simulink model "DoubleTankSim_NonLinearCtrl"  (R2025b)
settings: Solver=VariableStepAuto  StartTime=0.0  StopTime=1500  RelTol=1e-3
values from neighbouring files (symbols this model uses):
  a_1 = 0.15025    [LabC.m]
  a_2 = 0.15615    [LabC.m]
  At = 33    [LabC.m]
  g = 981    [LabC.m]
  h_0 = 3.2    [LabC.m]
  Kd = 2*omega_n    (= 0.666666666667)    [LabC.m]
  Ki = 0.00005    (= 5e-05)    [LabC.m]
  Kp = omega_n^2    (= 0.111111111111)    [LabC.m]
  Q = [variance 0 0 ... (first row only)    [LabC.m]
  R = 0.1    [LabC.m]
  Ts = 0.02    [LabC.m]
  variance = 1e-8    (= 1e-08)    [LabC.m]
libraries: simulink x4, slpidlib x1
settings Model: Creator=kaspe  LastModifiedBy=William

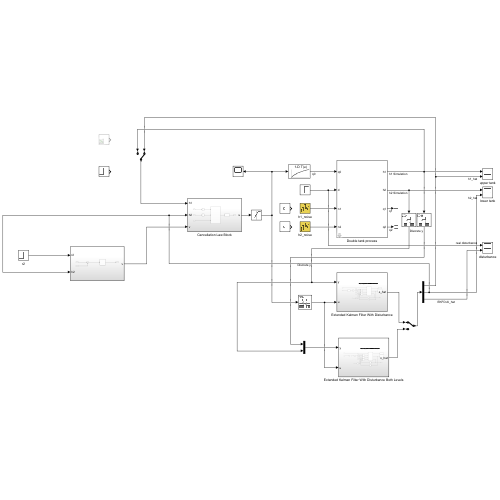
[thumbnail: Simulink's stored preview of the top-level diagram]
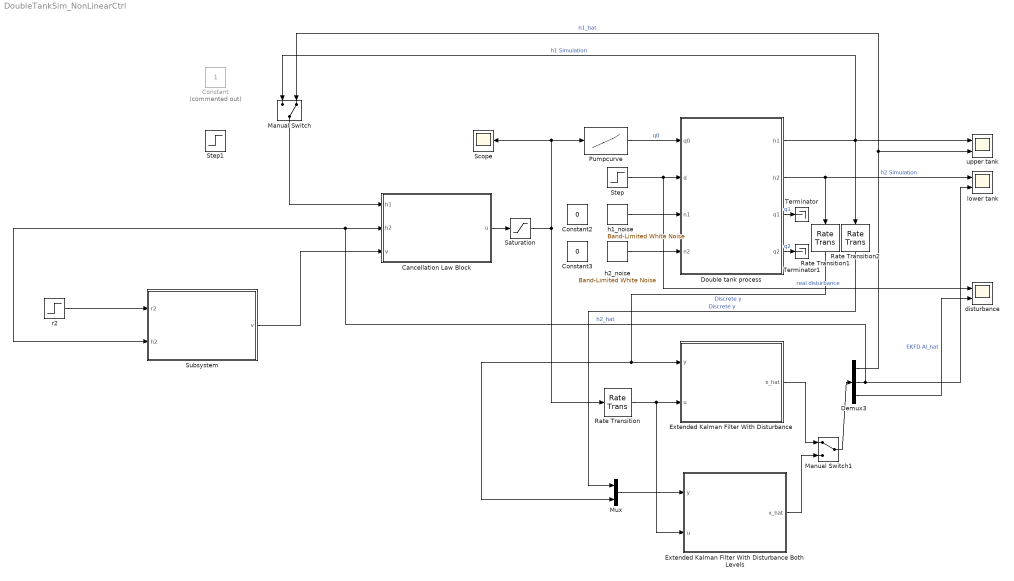
== system DoubleTankSim_NonLinearCtrl ==
  Cancellation Law Block : Subsystem
  Constant : Constant  Commented=on
  Constant2 : Constant  Value=0
  Constant3 : Constant  Value=0
  Demux3 : Demux  Outputs=3
  Double tank process : Subsystem  mask{At=33, a_1=0.151, a_2=0.16, hmax=15.5}
      mask prompts: At "Tank area (cm^2)"; a_1 "Upper tank opening area (cm^2)"; a_2 "Lower tank opening area (cm^2)"; hmax "Tank height (cm)"
      mask help: Double tank process parameters
  Extended Kalman Filter With Disturbance : Subsystem
  Extended Kalman Filter With Disturbance Both Levels : Subsystem
  Manual Switch : ManualSwitch  CurrentSetting=0
  Manual Switch1 : ManualSwitch
  Mux : Mux  Inputs=2
  Pumpcurve : Lookup_n-D  NumberOfTableDimensions=1  BreakpointsForDimension1=x  BreakpointsForDimension2=[1:3]  Table=y  RndMeth=Simplest  mask{x=[0.5,1,1.5,2,2.5,3,3.5,5,8,10], y=[16.47,20.75,24.52,27.63,30.06,32.49,34.80,40.28,48.24,52.43]}
      mask prompts: x "Values on x-axis"; y "Values on y-axis"
  Rate Transition : RateTransition  OutPortSampleTime=Ts
  Rate Transition1 : RateTransition  OutPortSampleTime=Ts
  Rate Transition2 : RateTransition  OutPortSampleTime=Ts
  Saturation : Saturate  UpperLimit=10  LowerLimit=0
  Scope : Scope
      settings: ActiveDisplayYMinimum=-1.2499999999999998  ActiveDisplayYMaximum=11.25  DataLoggingVariableName=ScopeData3
  Step : Step  Time=900  After=0.1  SampleTime=0
  Step1 : Step  Time=750  Before=1  After=1.25  SampleTime=0
  Subsystem : Subsystem
  Terminator : Terminator
  Terminator1 : Terminator
  disturbance : Scope  NumInputPorts=2
      settings: ActiveDisplayYMinimum=-1  ActiveDisplayYMaximum=1  DataLoggingVariableName=ScopeData2
  h1_noise : simulink/Sources/Band-Limited White Noise  Cov=[variance]  Ts=Ts  seed=[23342]
  h2_noise : simulink/Sources/Band-Limited White Noise  Cov=[variance]  Ts=Ts  seed=[23341]
  lower tank : Scope  NumInputPorts=2
      settings: ActiveDisplayYMinimum=-1.517228382859021  ActiveDisplayYMaximum=13.607589492730195
  r2 : Step  Time=500  Before=8  After=12  SampleTime=0
  upper tank : Scope  NumInputPorts=2
      settings: ActiveDisplayYMinimum=-1.986368348644401  ActiveDisplayYMaximum=17.525078273134039
  wires:
  Extended Kalman Filter With Disturbance/1(x_hat) -> Manual Switch1/1
  Pumpcurve/1 -> Double tank process/1(q0)  "q0"
  Double tank process/1(h1) -> upper tank/1, Manual Switch/1, Rate Transition2/1  "h1 Simulation"
  Step/1 -> Double tank process/2(d), disturbance/1  "real disturbance"
  h1_noise/1 -> Double tank process/3(n1)
  h2_noise/1 -> Double tank process/4(n2)
  Demux3/1 -> upper tank/2, Manual Switch/2  "h1_hat"
  Double tank process/2(h2) -> lower tank/1, Rate Transition1/1  "h2 Simulation"
  Demux3/2 -> Cancellation Law Block/2(h2), Subsystem/2(h2), lower tank/2  "h2_hat"
  Demux3/3 -> disturbance/2  "EKFD Al_hat"
  Rate Transition1/1 -> Extended Kalman Filter With Disturbance/1(y), Mux/2  "Discrete y"
  Rate Transition/1 -> Extended Kalman Filter With Disturbance/2(u), Extended Kalman Filter With Disturbance Both Levels/2(u)
  Double tank process/3(q1) -> Terminator/1  "q1"
  Double tank process/4(q2) -> Terminator1/1  "q2"
  Subsystem/1(v) -> Cancellation Law Block/3(v)
  Manual Switch/1 -> Cancellation Law Block/1(h1)
  r2/1 -> Subsystem/1(r2)
  Cancellation Law Block/1(u) -> Saturation/1
  Saturation/1 -> Scope/1, Pumpcurve/1, Rate Transition/1
  Mux/1 -> Extended Kalman Filter With Disturbance Both Levels/1(y)
  Rate Transition2/1 -> Mux/1  "Discrete y"
  Extended Kalman Filter With Disturbance Both Levels/1(x_hat) -> Manual Switch1/2
  Manual Switch1/1 -> Demux3/1

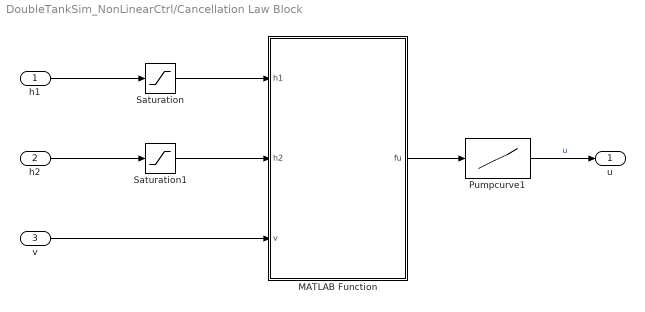
== system DoubleTankSim_NonLinearCtrl/Cancellation Law Block ==
  h1 : Inport
  h2 : Inport  Port=2
  v : Inport  Port=3
  MATLAB Function : MATLAB Function  TreatAsAtomicUnit=on
  Pumpcurve1 : Lookup_n-D  NumberOfTableDimensions=1  BreakpointsForDimension1=x  BreakpointsForDimension2=[1:3]  Table=y  RndMeth=Simplest  mask{x=[16.47,20.75,24.52,27.63,30.06,32.49,34.80,40.28,48.24,52.43], y=[0.5,1,1.5,2,2.5,3,3.5,5,8,10]}
      mask prompts: x "Values on x-axis"; y "Values on y-axis"
  Saturation : Saturate  UpperLimit=15.5  LowerLimit=0.001
  Saturation1 : Saturate  UpperLimit=15.5  LowerLimit=0.001
  u : Outport
  wires:
  MATLAB Function/1(fu) -> Pumpcurve1/1
  h1/1 -> Saturation/1
  h2/1 -> Saturation1/1
  Pumpcurve1/1 -> u/1  "u"
  v/1 -> MATLAB Function/3(v)
  Saturation/1 -> MATLAB Function/1(h1)
  Saturation1/1 -> MATLAB Function/2(h2)

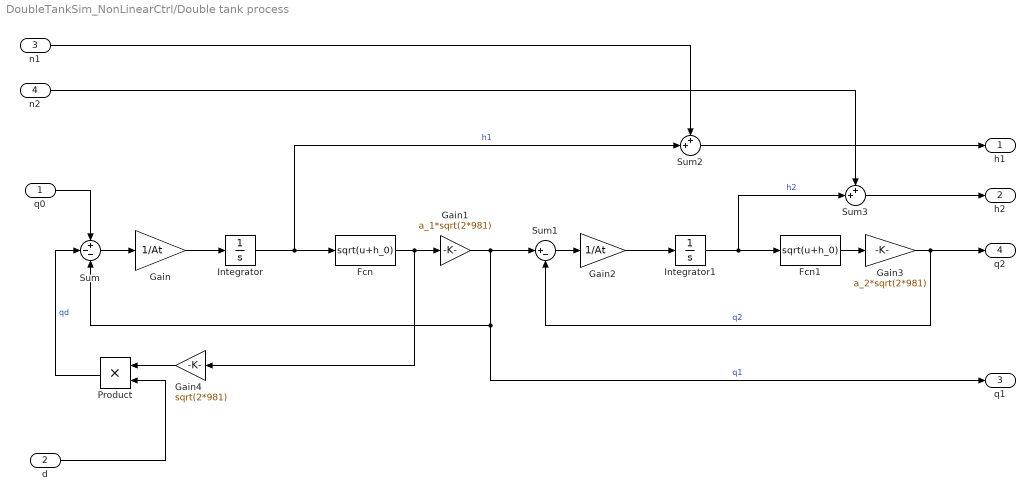
== system DoubleTankSim_NonLinearCtrl/Double tank process ==
  q0 : Inport
  d : Inport  Port=2
  n1 : Inport  Port=3
  n2 : Inport  Port=4
  Fcn : Fcn  Expr=sqrt(u+h_0)
  Fcn1 : Fcn  Expr=sqrt(u+h_0)
  Gain : Gain  Gain=1/At
  Gain1 : Gain  Gain=a_1*sqrt(2*981)
  Gain2 : Gain  Gain=1/At
  Gain3 : Gain  Gain=a_2*sqrt(2*981)
  Gain4 : Gain  Gain=sqrt(2*981)
  Integrator : Integrator  LimitOutput=on  UpperSaturationLimit=hmax  LowerSaturationLimit=0
  Integrator1 : Integrator  LimitOutput=on  UpperSaturationLimit=hmax  LowerSaturationLimit=0
  Product : Product  RndMeth=Zero
  Sum : Sum  Inputs=+--
  Sum1 : Sum  Inputs=|+-
  Sum2 : Sum  Inputs=++|
  Sum3 : Sum  Inputs=++|
  h1 : Outport  VectorParamsAs1DForOutWhenUnconnected=off
  h2 : Outport  Port=2  VectorParamsAs1DForOutWhenUnconnected=off
  q1 : Outport  Port=3  VectorParamsAs1DForOutWhenUnconnected=off
  q2 : Outport  Port=4  VectorParamsAs1DForOutWhenUnconnected=off
  wires:
  Sum/1 -> Gain/1
  Gain/1 -> Integrator/1
  Fcn/1 -> Gain4/1, Gain1/1
  Gain1/1 -> Sum1/1, q1/1, Sum/3  "q1"
  Sum1/1 -> Gain2/1
  Gain2/1 -> Integrator1/1
  Fcn1/1 -> Gain3/1
  Gain3/1 -> Sum1/2, q2/1  "q2"
  q0/1 -> Sum/1
  Integrator/1 -> Sum2/2, Fcn/1  "h1"
  Product/1 -> Sum/2  "qd"
  Integrator1/1 -> Sum3/2, Fcn1/1  "h2"
  d/1 -> Product/2
  Sum2/1 -> h1/1
  n1/1 -> Sum2/1
  Sum3/1 -> h2/1
  n2/1 -> Sum3/1
  Gain4/1 -> Product/1

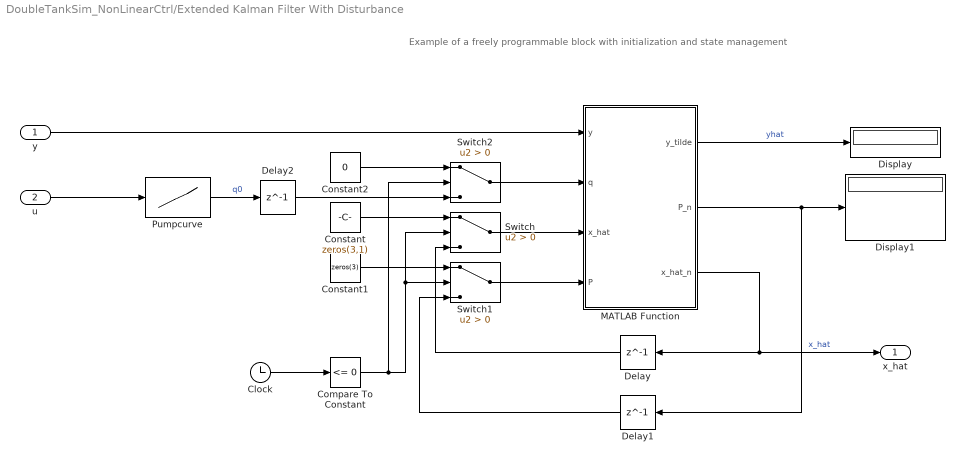
== system DoubleTankSim_NonLinearCtrl/Extended Kalman Filter With Disturbance ==
  note: Example of a freely programmable block with initialization and state management
  y : Inport
  u : Inport  Port=2
  Clock : Clock
  Compare To Constant : simulink/Logic and Bit Operations/Compare To Constant  relop=<=  const=0  OutDataTypeStr=boolean
  Constant : Constant  Value=zeros(3,1)
  Constant1 : Constant  Value=zeros(3)
  Constant2 : Constant  Value=0
  Delay : Delay  DelayLength=1  InitialCondition=0
  Delay1 : Delay  DelayLength=1  InitialCondition=0
  Delay2 : Delay  DelayLength=1  InitialCondition=0
  Display : Display
  Display1 : Display
  MATLAB Function : MATLAB Function  TreatAsAtomicUnit=on
  Pumpcurve : Lookup_n-D  NumberOfTableDimensions=1  BreakpointsForDimension1=x  BreakpointsForDimension2=[1:3]  Table=y  RndMeth=Simplest  mask{x=[0.5,1,1.5,2,2.5,3,3.5,5,8,10], y=[16.47,20.75,24.52,27.63,30.06,32.49,34.80,40.28,48.24,52.43]}
      mask prompts: x "Values on x-axis"; y "Values on y-axis"
  Switch : Switch  Criteria=u2 > Threshold  SaturateOnIntegerOverflow=off  InputSameDT=off
  Switch1 : Switch  Criteria=u2 > Threshold  SaturateOnIntegerOverflow=off  InputSameDT=off
  Switch2 : Switch  Criteria=u2 > Threshold  SaturateOnIntegerOverflow=off  InputSameDT=off
  x_hat : Outport  PortDimensions=3
  wires:
  Delay/1 -> Switch/3
  Switch/1 -> MATLAB Function/3(x_hat)
  Constant1/1 -> Switch1/1
  Compare To Constant/1 -> Switch2/2, Switch/2, Switch1/2
  Constant/1 -> Switch/1
  MATLAB Function/1(y_tilde) -> Display/1  "yhat"
  MATLAB Function/2(P_n) -> Delay1/1, Display1/1
  Clock/1 -> Compare To Constant/1
  Switch1/1 -> MATLAB Function/4(P)
  y/1 -> MATLAB Function/1(y)
  Delay1/1 -> Switch1/3
  Switch2/1 -> MATLAB Function/2(q)
  Constant2/1 -> Switch2/1
  Delay2/1 -> Switch2/3
  Pumpcurve/1 -> Delay2/1  "q0"
  u/1 -> Pumpcurve/1
  MATLAB Function/3(x_hat_n) -> Delay/1, x_hat/1  "x_hat"

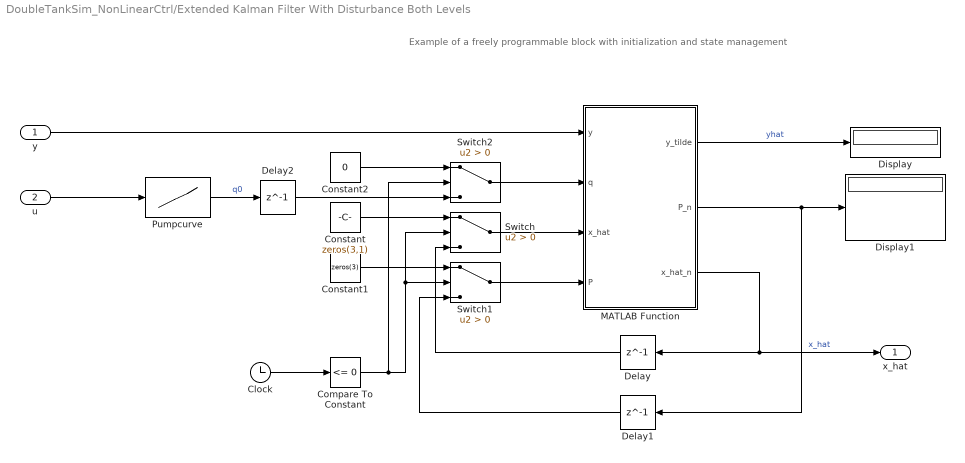
== system DoubleTankSim_NonLinearCtrl/Extended Kalman Filter With Disturbance Both Levels ==
  note: Example of a freely programmable block with initialization and state management
  y : Inport
  u : Inport  Port=2
  Clock : Clock
  Compare To Constant : simulink/Logic and Bit Operations/Compare To Constant  relop=<=  const=0  OutDataTypeStr=boolean
  Constant : Constant  Value=zeros(3,1)
  Constant1 : Constant  Value=zeros(3)
  Constant2 : Constant  Value=0
  Delay : Delay  DelayLength=1  InitialCondition=0
  Delay1 : Delay  DelayLength=1  InitialCondition=0
  Delay2 : Delay  DelayLength=1  InitialCondition=0
  Display : Display
  Display1 : Display
  MATLAB Function : MATLAB Function  TreatAsAtomicUnit=on
  Pumpcurve : Lookup_n-D  NumberOfTableDimensions=1  BreakpointsForDimension1=x  BreakpointsForDimension2=[1:3]  Table=y  RndMeth=Simplest  mask{x=[0.5,1,1.5,2,2.5,3,3.5,5,8,10], y=[16.47,20.75,24.52,27.63,30.06,32.49,34.80,40.28,48.24,52.43]}
      mask prompts: x "Values on x-axis"; y "Values on y-axis"
  Switch : Switch  Criteria=u2 > Threshold  SaturateOnIntegerOverflow=off  InputSameDT=off
  Switch1 : Switch  Criteria=u2 > Threshold  SaturateOnIntegerOverflow=off  InputSameDT=off
  Switch2 : Switch  Criteria=u2 > Threshold  SaturateOnIntegerOverflow=off  InputSameDT=off
  x_hat : Outport  PortDimensions=3
  wires:
  Delay/1 -> Switch/3
  Switch/1 -> MATLAB Function/3(x_hat)
  Constant1/1 -> Switch1/1
  Compare To Constant/1 -> Switch2/2, Switch/2, Switch1/2
  Constant/1 -> Switch/1
  MATLAB Function/1(y_tilde) -> Display/1  "yhat"
  MATLAB Function/2(P_n) -> Delay1/1, Display1/1
  Clock/1 -> Compare To Constant/1
  Switch1/1 -> MATLAB Function/4(P)
  y/1 -> MATLAB Function/1(y)
  Delay1/1 -> Switch1/3
  Switch2/1 -> MATLAB Function/2(q)
  Constant2/1 -> Switch2/1
  Delay2/1 -> Switch2/3
  Pumpcurve/1 -> Delay2/1  "q0"
  u/1 -> Pumpcurve/1
  MATLAB Function/3(x_hat_n) -> Delay/1, x_hat/1  "x_hat"

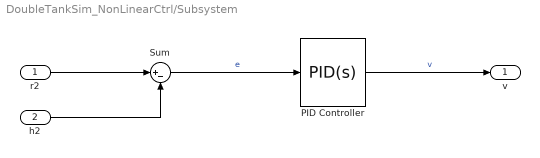
== system DoubleTankSim_NonLinearCtrl/Subsystem ==
  r2 : Inport
  h2 : Inport  Port=2
  PID Controller : slpidlib/PID Controller  Controller=PID  Form=Parallel  TimeDomain=Continuous-time  UseExternalTs=off  SampleTime=-1  IntegratorMethod=Forward Euler  FilterMethod=Forward Euler  ControllerParametersSource=internal  P=Kp  I=Ki  UseKiTs=off  D=Kd  UseExternalDerivativeSource=off  N=1  UseFilter=on  TunerSelectOption=Transfer Function Based (PID Tuner App)  InitialConditionSource=internal  InitialConditionForIntegrator=0  InitialConditionForFilter=0  DifferentiatorICPrevScaledInput=0  ExternalReset=none  TrackingMode=off  Kt=1  LimitOutput=off  SatLimitsSource=internal  UpperSaturationLimit=inf  LowerSaturationLimit=-inf  LinearizeAsGain=on  AntiWindupMode=none  Kb=1  LimitIntegrator=off  UpperIntegratorSaturationLimit=inf  LowerIntegratorSaturationLimit=-inf  POutMin=[]  POutMax=[]  IOutMin=[]  IOutMax=[]  DOutMin=[]  DOutMax=[]  NOutMin=[]  NOutMax=[]  SumOutMin=[]  SumOutMax=[]  SaturationOutMin=[]  SaturationOutMax=[]  PParamMin=[]  PParamMax=[]  IParamMin=[]  IParamMax=[]  DParamMin=[]  DParamMax=[]  NParamMin=[]  NParamMax=[]  KbParamMin=[]  KbParamMax=[]  KtParamMin=[]  KtParamMax=[]  KbOutMin=[]  KbOutMax=[]  KtOutMin=[]  KtOutMax=[]  IntegratorOutMin=[]  IntegratorOutMax=[]  FilterOutMin=[]  FilterOutMax=[]  SumI1OutMin=[]  SumI1OutMax=[]  SumI2OutMin=[]  SumI2OutMax=[]  SumI3OutMin=[]  SumI3OutMax=[]  SumI4OutMin=[]  SumI4OutMax=[]  SumDOutMin=[]  SumDOutMax=[]  DifferentiatorOutMin=[]  DifferentiatorOutMax=[]  FilterDiffOutCoefMin=[]  FilterDiffOutCoefMax=[]  ReciprocalOutMin=[]  ReciprocalOutMax=[]  SumDenOutMin=[]  SumDenOutMax=[]  SumNumOutMin=[]  SumNumOutMax=[]  DivideOutMin=[]  DivideOutMax=[]  UdiffTsProdOutMin=[]  UdiffTsProdOutMax=[]  NTsProdOutMin=[]  NTsProdOutMax=[]  UintegralTsProdOutMin=[]  UintegralTsProdOutMax=[]  UngainTsProdOutMin=[]  UngainTsProdOutMax=[]  ClampingZeroOutDataTypeStr=Inherit: Inherit via back propagation  ClampingZeroOutMin=[]  ClampingZeroOutMax=[]  FilterDenConstantOutDataTypeStr=Inherit: Inherit via back propagation  FilterDenConstantOutMin=[]  FilterDenConstantOutMax=[]  PCopyOutDataTypeStr=Inherit: Inherit via back propagation  PCopyOutMin=[]  PCopyOutMax=[]  NCopyOutDataTypeStr=Inherit: Inherit via back propagation  NCopyOutMin=[]  NCopyOutMax=[]  IntegratorContinuousStateAttributes=''  IntegratorStateMustResolveToSignalObject=off  IntegratorRTWStateStorageClass=Auto  FilterContinuousStateAttributes=''  FilterStateMustResolveToSignalObject=off  FilterRTWStateStorageClass=Auto  ParallelPVariant=InternalParameters  IdealPVariant=Disabled  IVariant=InternalParameters  DVariant=InternalParameters  IntegratorVariant=Continuous  SatVariant=Disabled  AWVariant=Passthrough  PCopyVariant=Disabled  TRVariant=Disabled  FdbkBlocksVariant=Forward  IdealPFdbkVariant=Disabled  SatFdbkVariant=Disabled  DerivativeFilterVariant=ContFilter  NVariant=InternalParameters  NCopyVariant=Disabled  FilterICVariant=InternalICsFilter  IntegratorICVariant=InternalICs  ExternalResetVariant=Disabled  TRSumVariant=Passthrough  SumFdbkVariant=Disabled  SumVariant=Sum_PID  TsampFilterVariant=InternalTs  TsampNgainVariant=Passthrough  TsampIntegralVariant=Disabled_SignalSpec  ExternalSaturationOutDataTypeStr=Inherit: Same as second input  DerivativeSourceVariant=ErrorSignal  PreIntVariant=InternalPreInt
  Sum : Sum  Inputs=|+-
  v : Outport
  wires:
  h2/1 -> Sum/2
  Sum/1 -> PID Controller/1  "e"
  PID Controller/1 -> v/1  "v"
  r2/1 -> Sum/1

== matlab function DoubleTankSim_NonLinearCtrl/Extended Kalman Filter With Disturbance Both Levels/MATLAB Function ==
  data: y input; q input; x_hat input; At parameter; a_1 parameter; a_2 parameter; h_0 parameter; y_tilde output; P input; P_n output; x_hat_n output; Q parameter; R parameter; g parameter; Ts parameter
function [y_tilde, P_n, x_hat_n] = fcn(y, q, x_hat, At, a_1, a_2, h_0, P, Q, R, g, Ts)

% Linearization
h_hat1 = x_hat(1);
h_hat2 = x_hat(2);
a_l = x_hat(3);

sqrt1 = sqrt(2*g*(max([h_hat1+h_0,0])));
sqrt2 = sqrt(2*g*(max([h_hat2+h_0,0])));

A = [-(a_1 + a_l)*g/At/sqrt1, 0,              -sqrt1/At;
     a_1*g/At/sqrt1,           -a_2*g/At/sqrt2, 0
     0,                       0,              0];

C = [1 0 0;
    0 1 0];

Ad = eye(size(A)) + Ts * A;

% Predict
x_hat_dot = [(q - (a_1 + a_l)*sqrt1)/At; 
             (a_1*sqrt1 - a_2*sqrt2)/At;
             0];
x_hat_n = x_hat + x_hat_dot .* Ts;
P_n = Ad * P * Ad' + Q;

R = diag([0.1, 0.1]);

% Update
y_tilde = y - C * x_hat_n;
S = C * P_n * C' + R;
K = P_n * C' * inv(S);
x_hat_n = x_hat_n + K * y_tilde;
P_n = (eye(size(A)) - K * C) * P_n;   
y_tilde = y - C * x_hat_n;

== matlab function DoubleTankSim_NonLinearCtrl/Cancellation Law Block/MATLAB Function ==
  data: h1 input; fu output; h2 input; v input; h_0 parameter; At parameter; a_1 parameter; a_2 parameter; g parameter
function fu = fcn(h1, h2, v, h_0, At, a_1, a_2, g)

% this function computes f(u) so that all the non-linear terms are canceled

q1 = sqrt(2*g*(h1 + h_0));  % ← Math Function block (sqrt), with Gain 2*g beforehand
q2 = sqrt(2*g*(h2 + h_0));  % ← same structure

phi = -(a_1^2*g/At^2) - (a_2*g*(a_1*q1 - a_2*q2))/(At^2*q2);

beta = (a_1*g) / (At^2*q1);

fu = (v - phi) / beta;

== matlab function DoubleTankSim_NonLinearCtrl/Extended Kalman Filter With Disturbance/MATLAB Function ==
  data: y input; q input; x_hat input; At parameter; a_1 parameter; a_2 parameter; h_0 parameter; y_tilde output; P input; P_n output; x_hat_n output; Q parameter; R parameter; g parameter; Ts parameter
function [y_tilde, P_n, x_hat_n] = fcn(y, q, x_hat, At, a_1, a_2, h_0, P, Q, R, g, Ts)

% Linearization
h_hat1 = x_hat(1);
h_hat2 = x_hat(2);
a_l = x_hat(3);

sqrt1 = sqrt(2*g*(max([h_hat1+h_0,0])));
sqrt2 = sqrt(2*g*(max([h_hat2+h_0,0])));

A = [-(a_1 + a_l)*g/At/sqrt1, 0,              -sqrt1/At;
     a_1*g/At/sqrt1,           -a_2*g/At/sqrt2, 0
     0,                       0,              0];

C = [0 1 0];

Ad = eye(size(A)) + Ts * A;

% Predict
x_hat_dot = [(q - (a_1 + a_l)*sqrt1)/At; 
             (a_1*sqrt1 - a_2*sqrt2)/At;
             0];
x_hat_n = x_hat + x_hat_dot .* Ts;
P_n = Ad * P * Ad' + Q;

% Update
y_tilde = y - C * x_hat_n;
S = C * P_n * C' + R;
K = P_n * C' * inv(S);
x_hat_n = x_hat_n + K * y_tilde;
P_n = (eye(size(A)) - K * C) * P_n;   
y_tilde = y - C * x_hat_n;
